simulink model "kinematicModel"  (R2014b)
settings: Solver=ode45  StartTime=0.0  StopTime=2000  RelTol=1e-3
libraries: simulink x1
settings Model: Creator=einagd  LastModifiedBy=einagd
settings DebuggingCC: SolverPrmCheckMsg=none

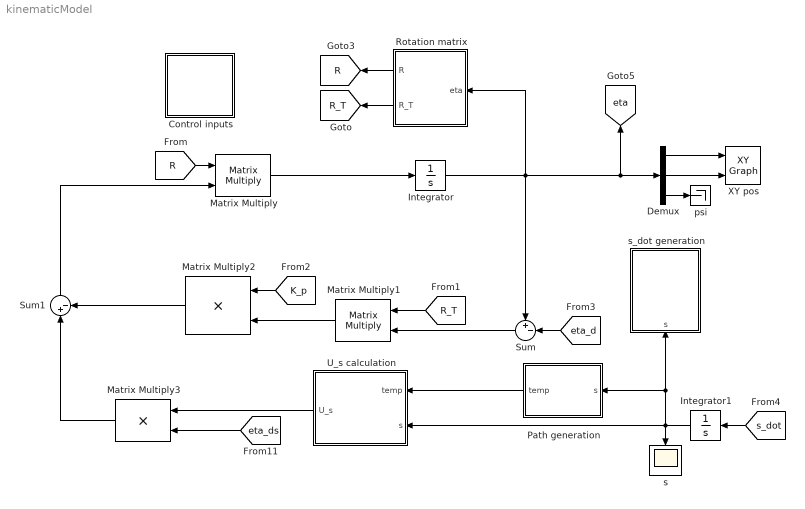
== system kinematicModel ==
  Control inputs : Subsystem
  Demux : Demux  Outputs=3
  Integrator : Integrator  InitialCondition=[7;0;0]
  Integrator1 : Integrator
  Matrix Multiply : Product  Multiplication=Matrix(*)
  Matrix Multiply1 : Product  Multiplication=Matrix(*)
  Matrix Multiply2 : Product
  Matrix Multiply3 : Product
  Path generation : Subsystem
  Rotation matrix : MATLAB Function  TreatAsAtomicUnit=on
  Sum : Sum  Inputs=+-|
  Sum1 : Sum  Inputs=|+-
  U_s calculation : Subsystem
  XY pos : simulink/Sinks/XY Graph  xmin=0  xmax=15  ymin=-5  ymax=5  st=-1
  psi : Terminator
  s : Scope
      settings: ShowLegends=on
  s_dot generation : Subsystem
  tag scope: R=global, R_T=global, eta=global
  wires:
  Integrator/1 -> Sum/1, Rotation matrix/1(eta), Demux/1, [eta]
  Matrix Multiply/1 -> Integrator/1
  Sum/1 -> Matrix Multiply1/2
  [R_T] -> Matrix Multiply1/1
  [s_dot] -> Integrator1/1
  Matrix Multiply2/1 -> Sum1/2
  Matrix Multiply3/1 -> Sum1/1
  Rotation matrix/2(R_T) -> [R_T]
  Rotation matrix/1(R) -> [R]
  [R] -> Matrix Multiply/1
  Sum1/1 -> Matrix Multiply/2
  [K_p] -> Matrix Multiply2/1
  Matrix Multiply1/1 -> Matrix Multiply2/2
  [eta_ds] -> Matrix Multiply3/2
  Demux/1 -> XY pos/1
  Demux/2 -> XY pos/2
  Demux/3 -> psi/1
  Path generation/1(temp) -> U_s calculation/1(temp)
  U_s calculation/1(U_s) -> Matrix Multiply3/1
  [eta_d] -> Sum/2
  Integrator1/1 -> s/1, Path generation/1(s), s_dot generation/1(s), U_s calculation/2(s)

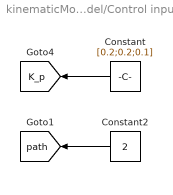
== system kinematicModel/Control inputs ==
  Constant : Constant  Value=[0.2;0.2;0.1]  VectorParams1D=off
  Constant2 : Constant  Value=2
  tag scope: K_p=global, path=global
  wires:
  Constant/1 -> [K_p]
  Constant2/1 -> [path]

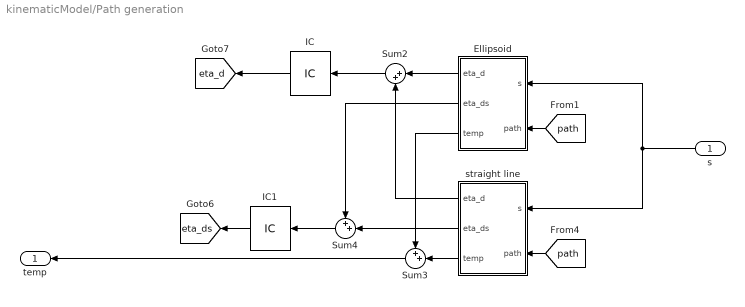
== system kinematicModel/Path generation ==
  s : Inport
  Ellipsoid : MATLAB Function  TreatAsAtomicUnit=on
  IC : InitialCondition  Value=[0;0;0]
  IC1 : InitialCondition  Value=[0.00001;0.00001;0.00001]
  Sum2 : Sum  Inputs=|++
  Sum3 : Sum  Inputs=++|
  Sum4 : Sum  Inputs=++|
  straight line : MATLAB Function  TreatAsAtomicUnit=on
  temp : Outport
  tag scope: eta_d=global, eta_ds=global
  wires:
  IC1/1 -> [eta_ds]
  Ellipsoid/2(eta_ds) -> Sum4/1
  Ellipsoid/3(temp) -> Sum3/1
  Sum3/1 -> temp/1
  [path] -> straight line/2(path)
  straight line/2(eta_ds) -> Sum4/2
  straight line/3(temp) -> Sum3/2
  Sum4/1 -> IC1/1
  Sum2/1 -> IC/1
  [path] -> Ellipsoid/2(path)
  Ellipsoid/1(eta_d) -> Sum2/1
  straight line/1(eta_d) -> Sum2/2
  IC/1 -> [eta_d]
  s/1 -> straight line/1(s), Ellipsoid/1(s)

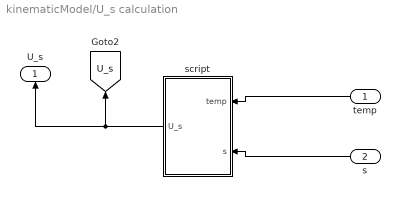
== system kinematicModel/U_s calculation ==
  temp : Inport
  s : Inport  Port=2
  script : MATLAB Function  TreatAsAtomicUnit=on
  U_s : Outport
  tag scope: U_s=global
  wires:
  script/1(U_s) -> U_s/1, [U_s]
  temp/1 -> script/1(temp)
  s/1 -> script/2(s)

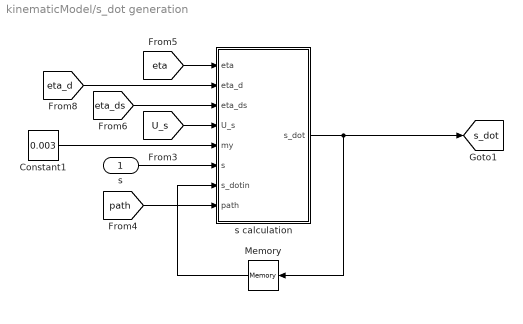
== system kinematicModel/s_dot generation ==
  s : Inport
  Constant1 : Constant  Value=0.003
  Memory : Memory  X0=0.0000001
  s calculation : MATLAB Function  TreatAsAtomicUnit=on
  tag scope: s_dot=global
  wires:
  [eta_d] -> s calculation/2(eta_d)
  [eta] -> s calculation/1(eta)
  s calculation/1(s_dot) -> Memory/1, [s_dot]
  [U_s] -> s calculation/4(U_s)
  Constant1/1 -> s calculation/5(my)
  Memory/1 -> s calculation/7(s_dotin)
  [eta_ds] -> s calculation/3(eta_ds)
  [path] -> s calculation/8(path)
  s/1 -> s calculation/6(s)

== matlab function kinematicModel/Path generation/straight line ==
  data: eta_d output; eta_ds output; temp output; s input; path input
function [eta_d,eta_ds,temp] = fcn(s,path)
%#codegen
x0 = 2;
y0 = 0;
x1 = 10;
y1 = 4;

a1 = x1-x0;
a2 = y1-y0;

xd = a1*s+x0;
yd = a2*s+y0;
psi_d = atan2(yd,xd);

eta_d = [xd;yd;psi_d]*(2-path);
eta_ds = [a1;a2;0]*(2-path);

temp = (1/(sqrt(a1^2+a2^2)))*(2-path);


end

== matlab function kinematicModel/Rotation matrix ==
  data: eta input; R output; R_T output
function [R,R_T] = fcn(eta)

psi = eta(3);

R = [cos(psi) -sin(psi) 0;sin(psi) cos(psi) 0;0 0 1];
R_T = R';

end

== matlab function kinematicModel/s_dot generation/s calculation ==
  data: eta input; s_dot output; eta_d input; eta_ds input; U_s input; my input; s input; s_dotin input; path input
function s_dot = fcn(eta,eta_d,eta_ds,U_s,my,s,s_dotin,path)
%#codegen

%V_1s = -0.5*(eta_ds.')*(eta-eta_d)-0.5*((eta-eta_d).')*eta_ds;
V_1s = -((eta-eta_d).')*eta_ds;

s_dot = U_s - (my/norm(eta_ds))*V_1s;

if path == 1
    if s < 1 && s > 0
        if sign(s) == sign(s_dotin)
            s_dot = s_dot;
        else
            s_dot = s_dot*sign(s_dotin);
        end
    elseif s >= 1
        if sign(s) == sign(s_dotin)
            s_dot = -s_dot;
        else
            s_dot = s_dot*sign(s_dotin);
        end

    elseif s <= 0
        if sign(s) == sign(s_dotin)
            s_dot = s_dot;
        else
            s_dot = s_dot*sign(s_dotin);
        end
    end    
end
end

== matlab function kinematicModel/U_s calculation/script ==
  data: temp input; U_s output; s input
function U_s  = fcn(temp,s)

U_ref = 0.1;

U_s = temp*U_ref;

end

== matlab function kinematicModel/Path generation/Ellipsoid ==
  data: eta_d output; eta_ds output; temp output; s input; path input
function [eta_d,eta_ds,temp] = fcn(s,path)
rx = 5;
ry = 3;
cx = 6;
cy = 0;

xd = rx*cos(s) + cx;
yd = ry*sin(s) + cy;
psi_d = atan2(yd,xd);

xds = -rx*sin(s);
yds = ry*cos(s);
psi_ds = (rx*ry)/((rx*sin(s))^2+(ry*cos(s))^2);

eta_d = [xd;yd;psi_d]*(path-1);
eta_ds = [xds;yds;psi_ds]*(path-1);

temp = (1/(sqrt(xds^2+yds^2)))*(path-1);


end
